simulink model "step_response"  (R2021b)
settings: Solver=VariableStepAuto  StartTime=0.0  StopTime=13750.0  RelTol=1e-3
settings Model: Creator=Tino  LastModifiedBy=Tino

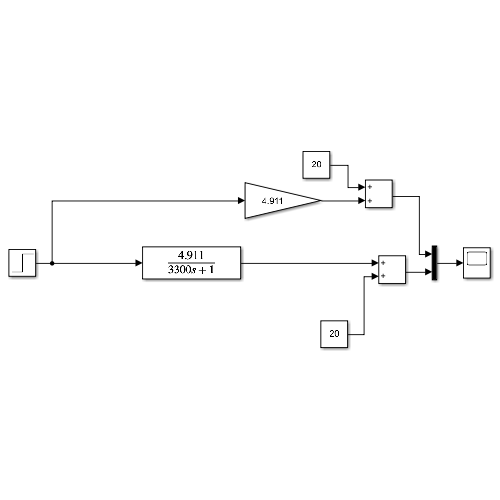
[thumbnail: Simulink's stored preview of the top-level diagram]
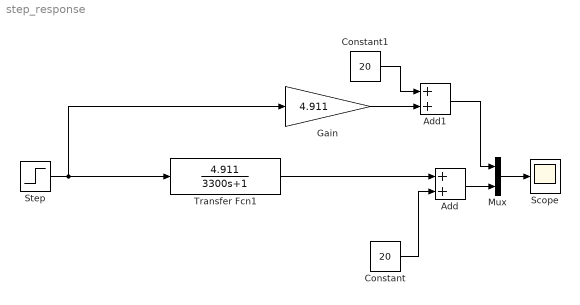
== system step_response ==
  Add : Sum
  Add1 : Sum
  Constant : Constant  Value=20
  Constant1 : Constant  Value=20
  Gain : Gain  Gain=4.911
  Mux : Mux  Inputs=2
  Scope : Scope
  Step : Step  After=17  SampleTime=0
  Transfer Fcn1 : TransferFcn  Numerator=[4.911]  Denominator=[3300 1]
  wires:
  Step/1 -> Transfer Fcn1/1, Gain/1
  Transfer Fcn1/1 -> Add/1
  Constant/1 -> Add/2
  Add/1 -> Mux/2
  Mux/1 -> Scope/1
  Add1/1 -> Mux/1
  Gain/1 -> Add1/2
  Constant1/1 -> Add1/1
